simulink model "controlSystem"  (R2023a)
settings: Solver=FixedStepDiscrete  StartTime=0.0  StopTime=inf  FixedStep=T  RelTol=1e-3  EnableMultiTasking=on
PreLoadFcn:
  | T=0.01;
  | alpha=0.02;
undefined symbols (not defined in the file): DiscIntNeverNeededParam
libraries: arduinolib x2, slpidlib x2, spsFirstOrderFilterLib x1, simulink x1, arduinosensorlib x1, arduinowifilib x1
settings Model: ExtModeTrigDuration=2  Creator=michele  LastModifiedBy=root
settings SolverCC: AlgebraicLoopSolver=TrustRegion
settings OptimizationCC: EnhancedBackFolding=on  PassReuseOutputArgsAs=Individual arguments  ZeroExternalMemoryAtStartup=off  ZeroInternalMemoryAtStartup=off  MaxStackSize=64  OptimizeBlockOrder=speed  DifferentSizesBufferReuse=on  OptimizationCustomize=off  EfficientTunableParamExpr=on
settings DebuggingCC: ParameterTunabilityLossMsg=error
settings HardwareCC: ProdBitPerPointer=32  ProdBitPerSizeT=32  ProdBitPerPtrDiffT=32  ProdLargestAtomicInteger=Long  ProdLargestAtomicFloat=Double  ProdWordSize=32  ProdHWDeviceType=ARM Compatible->ARM Cortex  UseEmbeddedCoderFeatures=off  UseSimulinkCoderFeatures=off
settings SFSimCC: MATLABDynamicMemAlloc=off
settings RTWCC: Description=Embedded Coder  SystemTargetFile=ert.tlc  HardwareBoard=ESP32-WROOM(Arduino Compatible)  TLCOptions="-aInlineSetEventsForThisBaseRateFcn=TLC_FALSE -aSuppressMultiTaskScheduler=TLC_FALSE  -aRateBasedStepFcn=0"  TemplateMakefile=ert_default_tmf  Toolchain=ESP32  BuildConfiguration=Faster Runs  DLArmComputeVersion=19.05
settings CodeAppCC: ForceParamTrailComments=on  IgnoreCustomStorageClasses=off  OperatorAnnotations=on  SimulinkDataObjDesc=on  SFDataObjDesc=on  MangleLength=10  InsertBlockDesc=on
settings ERTTargetCC: SupportContinuousTime=on  SupportNonInlinedSFcns=on  SupportVariableSizeSignals=on  ExtModeTransport=3  ExtModeStaticAlloc=on  ExtModeAutomaticAllocSize=off  ExtModeStaticAllocSize=65536  ExtModeMexFile=ext_xcp  ExtModeIntrfLevel=Level2 - Open

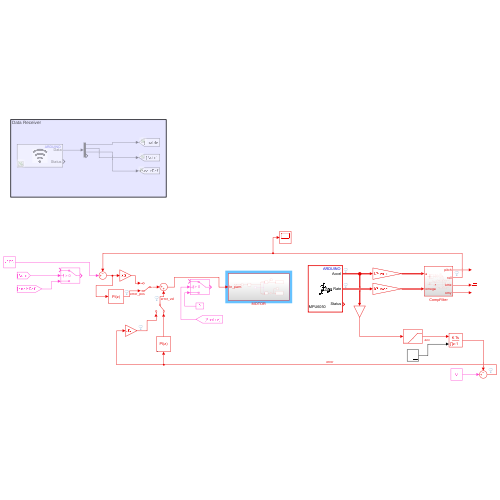
[thumbnail: Simulink's stored preview of the top-level diagram]
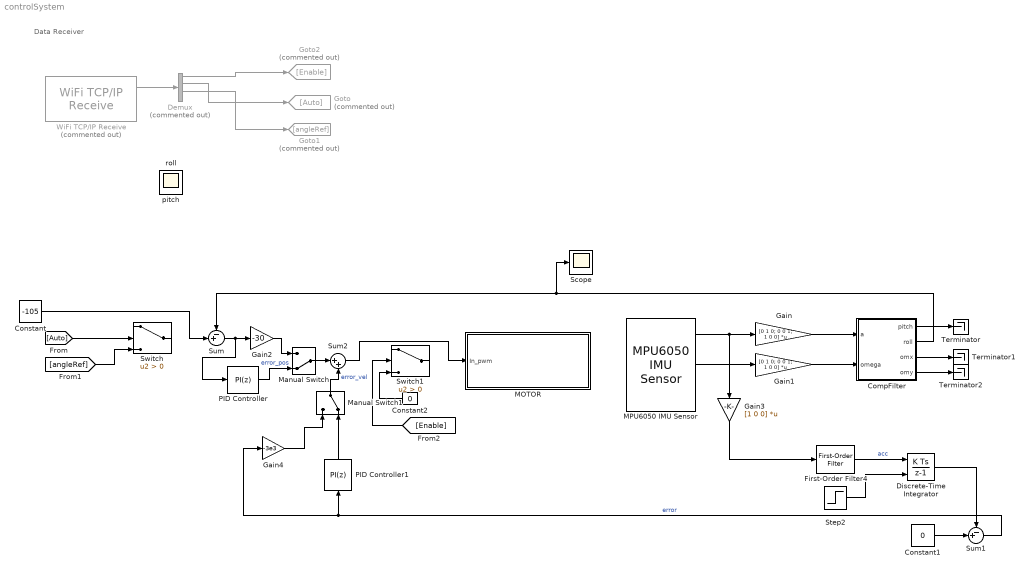
== system controlSystem ==
  note: Data Receiver
  CompFilter : Subsystem
  Constant : Constant  Value=-105
  Constant1 : Constant  Value=0
  Constant2 : Constant  Value=0
  Demux : Demux  Commented=on
  Discrete-Time Integrator : DiscreteIntegrator  ExternalReset=level  SampleTime=-1  ICPrevOutput=DiscIntNeverNeededParam  ICPrevScaledInput=DiscIntNeverNeededParam
  First-Order Filter4 : spsFirstOrderFilterLib/First-Order Filter  FilterType=Highpass  Tc=10e-3  Ts=0.01  Initialize=off  Vac_Init=[0, 0, 60]  Vdc_Init=0  PlotResponse=off  FreqRange="[0,  200,  1]"
  Gain : Gain  Gain=[0 1 0; 0 0 1; 1 0 0]  Multiplication=Matrix(K*u) (u vector)
  Gain1 : Gain  Gain=[0 1 0; 0 0 1; 1 0 0]  Multiplication=Matrix(K*u) (u vector)
  Gain2 : Gain  Gain=-30
  Gain3 : Gain  Gain=[1 0 0]  Multiplication=Matrix(K*u) (u vector)
  Gain4 : Gain  Gain=-3e3
  Goto : Goto  Commented=on  GotoTag=Auto
  Goto1 : Goto  Commented=on  GotoTag=angleRef
  Goto2 : Goto  Commented=on  GotoTag=Enable
  MOTOR : Subsystem
  MPU6050 IMU Sensor : arduinosensorlib/MPU6050 IMU Sensor  SlaveAddress=0x68  Accel=on  AngularRate=on  Temperature=off  Status=on  Timestamp=off  EulerAngles=off  Quat=off  AccelRange=2G  GyroRange=250 dps  DmpOdr=200 Hz  Dlpf=Accelerometer: 44Hz, Gyroscope: 42Hz  spf=1  SampleTime=-1  QueueSizeFactor=1
  Manual Switch : ManualSwitch  CurrentSetting=0
  Manual Switch1 : ManualSwitch  CurrentSetting=0
  PID Controller : slpidlib/PID Controller  Controller=PI  Form=Parallel  TimeDomain=Discrete-time  UseExternalTs=off  SampleTime=-1  IntegratorMethod=Forward Euler  FilterMethod=Forward Euler  ControllerParametersSource=internal  P=-4  I=-.3  UseKiTs=off  D=0  N=100  UseFilter=on  TunerSelectOption=Transfer Function Based (PID Tuner App)  InitialConditionSource=internal  InitialConditionForIntegrator=0  InitialConditionForFilter=0  DifferentiatorICPrevScaledInput=0  ExternalReset=none  TrackingMode=off  Kt=1  LimitOutput=off  SatLimitsSource=internal  UpperSaturationLimit=inf  LowerSaturationLimit=-inf  LinearizeAsGain=on  AntiWindupMode=none  Kb=1  LimitIntegrator=off  UpperIntegratorSaturationLimit=inf  LowerIntegratorSaturationLimit=-inf  POutMin=[]  POutMax=[]  IOutMin=[]  IOutMax=[]  DOutMin=[]  DOutMax=[]  NOutMin=[]  NOutMax=[]  SumOutMin=[]  SumOutMax=[]  SaturationOutMin=[]  SaturationOutMax=[]  PParamMin=[]  PParamMax=[]  IParamMin=[]  IParamMax=[]  DParamMin=[]  DParamMax=[]  NParamMin=[]  NParamMax=[]  KbParamMin=[]  KbParamMax=[]  KtParamMin=[]  KtParamMax=[]  KbOutMin=[]  KbOutMax=[]  KtOutMin=[]  KtOutMax=[]  IntegratorOutMin=[]  IntegratorOutMax=[]  FilterOutMin=[]  FilterOutMax=[]  SumI1OutMin=[]  SumI1OutMax=[]  SumI2OutMin=[]  SumI2OutMax=[]  SumI3OutMin=[]  SumI3OutMax=[]  SumI4OutMin=[]  SumI4OutMax=[]  SumDOutMin=[]  SumDOutMax=[]  DifferentiatorOutMin=[]  DifferentiatorOutMax=[]  FilterDiffOutCoefMin=[]  FilterDiffOutCoefMax=[]  ReciprocalOutMin=[]  ReciprocalOutMax=[]  SumDenOutMin=[]  SumDenOutMax=[]  SumNumOutMin=[]  SumNumOutMax=[]  DivideOutMin=[]  DivideOutMax=[]  UdiffTsProdOutMin=[]  UdiffTsProdOutMax=[]  NTsProdOutMin=[]  NTsProdOutMax=[]  UintegralTsProdOutMin=[]  UintegralTsProdOutMax=[]  UngainTsProdOutMin=[]  UngainTsProdOutMax=[]  ClampingZeroOutDataTypeStr=Inherit: Inherit via back propagation  ClampingZeroOutMin=[]  ClampingZeroOutMax=[]  FilterDenConstantOutDataTypeStr=Inherit: Inherit via back propagation  FilterDenConstantOutMin=[]  FilterDenConstantOutMax=[]  PCopyOutDataTypeStr=Inherit: Inherit via back propagation  PCopyOutMin=[]  PCopyOutMax=[]  NCopyOutDataTypeStr=Inherit: Inherit via back propagation  NCopyOutMin=[]  NCopyOutMax=[]  IntegratorContinuousStateAttributes=''  IntegratorStateMustResolveToSignalObject=off  IntegratorRTWStateStorageClass=Auto  FilterContinuousStateAttributes=''  FilterStateMustResolveToSignalObject=off  FilterRTWStateStorageClass=Auto  ParallelPVariant=InternalParameters  IdealPVariant=Disabled  IVariant=InternalParameters  DVariant=Disabled  IntegratorVariant=Discrete  SatVariant=Disabled  AWVariant=Passthrough  PCopyVariant=Disabled  TRVariant=Disabled  FdbkBlocksVariant=Forward  IdealPFdbkVariant=Disabled  SatFdbkVariant=Disabled  DerivativeFilterVariant=Disabled  NVariant=Disabled  NCopyVariant=Disabled_SignalSpec  FilterICVariant=Disabled  IntegratorICVariant=InternalICs  ExternalResetVariant=Disabled  TRSumVariant=Passthrough  SumFdbkVariant=Disabled  SumVariant=Sum_PI  TsampFilterVariant=InternalTs  TsampNgainVariant=Passthrough  TsampIntegralVariant=Disabled_SignalSpec  ExternalSaturationOutDataTypeStr=Inherit: Same as second input
  PID Controller1 : slpidlib/PID Controller  Controller=PI  Form=Parallel  TimeDomain=Discrete-time  UseExternalTs=off  SampleTime=-1  IntegratorMethod=Forward Euler  FilterMethod=Forward Euler  ControllerParametersSource=internal  P=-2e3  I=-3e2  UseKiTs=off  D=0  N=100  UseFilter=on  TunerSelectOption=Transfer Function Based (PID Tuner App)  InitialConditionSource=internal  InitialConditionForIntegrator=0  InitialConditionForFilter=0  DifferentiatorICPrevScaledInput=0  ExternalReset=none  TrackingMode=off  Kt=1  LimitOutput=off  SatLimitsSource=internal  UpperSaturationLimit=inf  LowerSaturationLimit=-inf  LinearizeAsGain=on  AntiWindupMode=none  Kb=1  LimitIntegrator=off  UpperIntegratorSaturationLimit=inf  LowerIntegratorSaturationLimit=-inf  POutMin=[]  POutMax=[]  IOutMin=[]  IOutMax=[]  DOutMin=[]  DOutMax=[]  NOutMin=[]  NOutMax=[]  SumOutMin=[]  SumOutMax=[]  SaturationOutMin=[]  SaturationOutMax=[]  PParamMin=[]  PParamMax=[]  IParamMin=[]  IParamMax=[]  DParamMin=[]  DParamMax=[]  NParamMin=[]  NParamMax=[]  KbParamMin=[]  KbParamMax=[]  KtParamMin=[]  KtParamMax=[]  KbOutMin=[]  KbOutMax=[]  KtOutMin=[]  KtOutMax=[]  IntegratorOutMin=[]  IntegratorOutMax=[]  FilterOutMin=[]  FilterOutMax=[]  SumI1OutMin=[]  SumI1OutMax=[]  SumI2OutMin=[]  SumI2OutMax=[]  SumI3OutMin=[]  SumI3OutMax=[]  SumI4OutMin=[]  SumI4OutMax=[]  SumDOutMin=[]  SumDOutMax=[]  DifferentiatorOutMin=[]  DifferentiatorOutMax=[]  FilterDiffOutCoefMin=[]  FilterDiffOutCoefMax=[]  ReciprocalOutMin=[]  ReciprocalOutMax=[]  SumDenOutMin=[]  SumDenOutMax=[]  SumNumOutMin=[]  SumNumOutMax=[]  DivideOutMin=[]  DivideOutMax=[]  UdiffTsProdOutMin=[]  UdiffTsProdOutMax=[]  NTsProdOutMin=[]  NTsProdOutMax=[]  UintegralTsProdOutMin=[]  UintegralTsProdOutMax=[]  UngainTsProdOutMin=[]  UngainTsProdOutMax=[]  ClampingZeroOutDataTypeStr=Inherit: Inherit via back propagation  ClampingZeroOutMin=[]  ClampingZeroOutMax=[]  FilterDenConstantOutDataTypeStr=Inherit: Inherit via back propagation  FilterDenConstantOutMin=[]  FilterDenConstantOutMax=[]  PCopyOutDataTypeStr=Inherit: Inherit via back propagation  PCopyOutMin=[]  PCopyOutMax=[]  NCopyOutDataTypeStr=Inherit: Inherit via back propagation  NCopyOutMin=[]  NCopyOutMax=[]  IntegratorContinuousStateAttributes=''  IntegratorStateMustResolveToSignalObject=off  IntegratorRTWStateStorageClass=Auto  FilterContinuousStateAttributes=''  FilterStateMustResolveToSignalObject=off  FilterRTWStateStorageClass=Auto  ParallelPVariant=InternalParameters  IdealPVariant=Disabled  IVariant=InternalParameters  DVariant=Disabled  IntegratorVariant=Discrete  SatVariant=Disabled  AWVariant=Passthrough  PCopyVariant=Disabled  TRVariant=Disabled  FdbkBlocksVariant=Forward  IdealPFdbkVariant=Disabled  SatFdbkVariant=Disabled  DerivativeFilterVariant=Disabled  NVariant=Disabled  NCopyVariant=Disabled_SignalSpec  FilterICVariant=Disabled  IntegratorICVariant=InternalICs  ExternalResetVariant=Disabled  TRSumVariant=Passthrough  SumFdbkVariant=Disabled  SumVariant=Sum_PI  TsampFilterVariant=InternalTs  TsampNgainVariant=Passthrough  TsampIntegralVariant=Disabled_SignalSpec  ExternalSaturationOutDataTypeStr=Inherit: Same as second input
  Scope : Scope
  Step2 : Step  Time=2  Before=1  After=0  SampleTime=0
  Sum : Sum  Inputs=-+|
  Sum1 : Sum  Inputs=-+|
  Sum2 : Sum  Inputs=|++
  Switch : Switch  Criteria=u2 > Threshold  SaturateOnIntegerOverflow=off  InputSameDT=off
  Switch1 : Switch  Criteria=u2 > Threshold  SaturateOnIntegerOverflow=off  InputSameDT=off
  Terminator : Terminator
  Terminator1 : Terminator
  Terminator2 : Terminator
  WiFi TCP/IP Receive : arduinowifilib/WiFi TCP//IP Receive  Commented=on  Mode_=Server  serverport=25000  RemoteAddr_=192.168.1.2  RemoteServerPort_=25000  DataType_=uint8  DataSize_=1  SampleTime_=0.1  remoteipoctet1=192  remoteipoctet2=168  remoteipoctet3=1  remoteipoctet4=2  wifiTCPServerIndex=0  wifiTCPClientIndex=0  blockPlatform=ARDUINO  isARMArch=false  SimulateUsing=Code generation  BlockingMode_=off  BlockTimeout_=0.1
  pitch : Scope
  roll : Scope
  wires:
  MPU6050 IMU Sensor/2 -> Gain1/1
  CompFilter/1(pitch) -> Terminator/1
  CompFilter/2(roll) -> Scope/1, Sum/1
  CompFilter/3(omx) -> Terminator1/1
  CompFilter/4(omy) -> Terminator2/1
  Gain/1 -> CompFilter/1(a)
  Gain1/1 -> CompFilter/2(omega)
  Gain2/1 -> Manual Switch/1
  Sum/1 -> PID Controller/1, Gain2/1
  PID Controller/1 -> Manual Switch/2  "error_pos"
  MPU6050 IMU Sensor/1 -> Gain/1, Gain3/1
  Discrete-Time Integrator/1 -> Sum1/1
  Step2/1 -> Discrete-Time Integrator/2
  First-Order Filter4/1 -> Discrete-Time Integrator/1  "acc"
  Gain3/1 -> First-Order Filter4/1
  Constant1/1 -> Sum1/2
  Sum1/1 -> Gain4/1, PID Controller1/1  "error"
  Manual Switch1/1 -> Sum2/2  "error_vel"
  Manual Switch/1 -> Sum2/1
  PID Controller1/1 -> Manual Switch1/2
  Gain4/1 -> Manual Switch1/1
  [Auto] -> Switch/2
  [angleRef] -> Switch/3
  Demux/3 -> Goto1/1
  WiFi TCP/IP Receive/1 -> Demux/1
  Demux/1 -> Goto2/1
  Demux/2 -> Goto/1
  Constant2/1 -> Switch1/3
  [Enable] -> Switch1/2
  Sum2/1 -> MOTOR/1(In_pwm)
  Constant/1 -> Sum/2

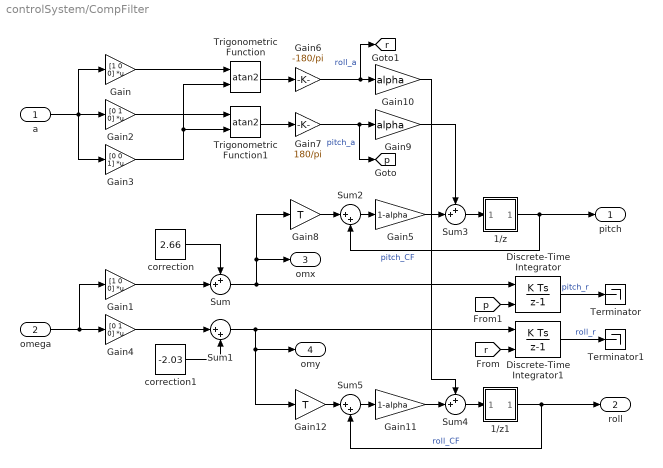
== system controlSystem/CompFilter ==
  a : Inport
  omega : Inport  Port=2
  1/z : Subsystem
  1/z1 : Subsystem
  Discrete-Time Integrator : DiscreteIntegrator  InitialConditionSource=external  SampleTime=-1  ICPrevOutput=DiscIntNeverNeededParam  ICPrevScaledInput=DiscIntNeverNeededParam
  Discrete-Time Integrator1 : DiscreteIntegrator  InitialConditionSource=external  SampleTime=-1  ICPrevOutput=DiscIntNeverNeededParam  ICPrevScaledInput=DiscIntNeverNeededParam
  Gain : Gain  Gain=[1 0 0]  Multiplication=Matrix(K*u)
  Gain1 : Gain  Gain=[1 0 0]  Multiplication=Matrix(K*u)
  Gain10 : Gain  Gain=alpha
  Gain11 : Gain  Gain=1-alpha
  Gain12 : Gain  Gain=T
  Gain2 : Gain  Gain=[0 1 0]  Multiplication=Matrix(K*u)
  Gain3 : Gain  Gain=[0 0 1]  Multiplication=Matrix(K*u)
  Gain4 : Gain  Gain=[0 1 0]  Multiplication=Matrix(K*u)
  Gain5 : Gain  Gain=1-alpha
  Gain6 : Gain  Gain=-180/pi
  Gain7 : Gain  Gain=180/pi
  Gain8 : Gain  Gain=T
  Gain9 : Gain  Gain=alpha
  Sum : Sum  Inputs=++|
  Sum1 : Sum  Inputs=|++
  Sum2 : Sum  Inputs=|++
  Sum3 : Sum  Inputs=++|
  Sum4 : Sum  Inputs=++|
  Sum5 : Sum  Inputs=|++
  Terminator : Terminator
  Terminator1 : Terminator
  Trigonometric Function : Trigonometry  Operator=atan2
  Trigonometric Function1 : Trigonometry  Operator=atan2
  correction : Constant  Value=2.66  SampleTime=T
  correction1 : Constant  Value=-2.03  SampleTime=T
  pitch : Outport
  roll : Outport  Port=2
  omx : Outport  Port=3
  omy : Outport  Port=4
  tag scope: p=global, r=global
  wires:
  a/1 -> Gain3/1, Gain2/1, Gain/1
  omega/1 -> Gain1/1, Gain4/1
  Trigonometric Function/1 -> Gain6/1
  Gain/1 -> Trigonometric Function/1
  Gain2/1 -> Trigonometric Function1/1
  Gain3/1 -> Trigonometric Function1/2, Trigonometric Function/2
  Trigonometric Function1/1 -> Gain7/1
  Discrete-Time Integrator1/1 -> Terminator1/1  "roll_r"
  Gain1/1 -> Sum/2
  Sum/1 -> Gain8/1, omx/1, Discrete-Time Integrator/1
  correction/1 -> Sum/1
  Gain4/1 -> Sum1/1
  correction1/1 -> Sum1/2
  Gain7/1 -> [p], Gain9/1  "pitch_a"
  Gain6/1 -> [r], Gain10/1  "roll_a"
  Sum2/1 -> Gain5/1
  Gain8/1 -> Sum2/1
  Gain9/1 -> Sum3/1
  1/z/1(out) -> pitch/1, Sum2/2  "pitch_CF"
  Gain5/1 -> Sum3/2
  Sum3/1 -> 1/z/1(in)
  Discrete-Time Integrator/1 -> Terminator/1  "pitch_r"
  1/z1/1(out) -> Sum5/2, roll/1  "roll_CF"
  Sum4/1 -> 1/z1/1(in)
  Gain11/1 -> Sum4/2
  Gain10/1 -> Sum4/1
  Sum1/1 -> omy/1, Gain12/1, Discrete-Time Integrator1/1
  Gain12/1 -> Sum5/1
  Sum5/1 -> Gain11/1
  [r] -> Discrete-Time Integrator1/2
  [p] -> Discrete-Time Integrator/2

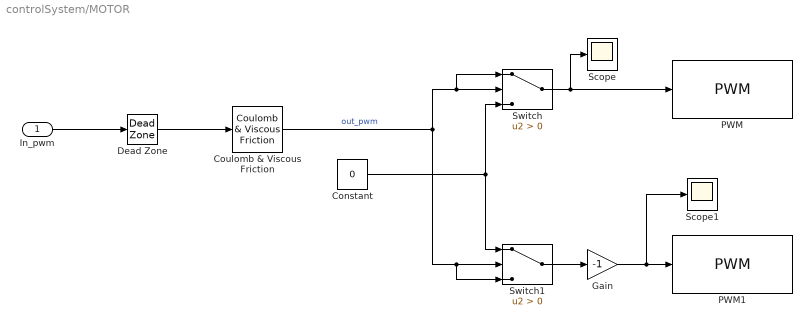
== system controlSystem/MOTOR ==
  In_pwm : Inport
  Constant : Constant  Value=0
  Coulomb & Viscous Friction : simulink/Discontinuities/Coulomb & Viscous Friction  offset=[180]  gain=1
  Dead Zone : DeadZone  LowerValue=-100  UpperValue=100
  Gain : Gain  Gain=-1
  PWM : arduinolib/PWM  pinNumber=32  frequencyType=Default  desiredFrequency=490.2  achievableFrequency=490.2
  PWM1 : arduinolib/PWM  pinNumber=33  frequencyType=Default  desiredFrequency=490.2  achievableFrequency=490.2
  Scope : Scope
  Scope1 : Scope
  Switch : Switch  Criteria=u2 > Threshold  SaturateOnIntegerOverflow=off  InputSameDT=off
  Switch1 : Switch  Criteria=u2 > Threshold  SaturateOnIntegerOverflow=off  InputSameDT=off
  wires:
  Switch1/1 -> Gain/1
  Gain/1 -> PWM1/1, Scope1/1
  Switch/1 -> Scope/1, PWM/1
  Constant/1 -> Switch1/1, Switch/3
  In_pwm/1 -> Dead Zone/1
  Coulomb & Viscous Friction/1 -> Switch1/2, Switch1/3, Switch/1, Switch/2  "out_pwm"
  Dead Zone/1 -> Coulomb & Viscous Friction/1

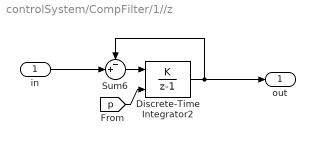
== system controlSystem/CompFilter/1//z ==
  in : Inport
  Discrete-Time Integrator2 : DiscreteIntegrator  IntegratorMethod=Accumulation: Forward Euler  InitialConditionSource=external  SampleTime=-1  ICPrevOutput=DiscIntNeverNeededParam  ICPrevScaledInput=DiscIntNeverNeededParam
  Sum6 : Sum  Inputs=-+|
  out : Outport
  wires:
  in/1 -> Sum6/2
  [p] -> Discrete-Time Integrator2/2
  Sum6/1 -> Discrete-Time Integrator2/1
  Discrete-Time Integrator2/1 -> out/1, Sum6/1

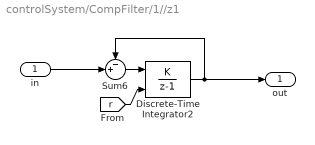
== system controlSystem/CompFilter/1//z1 ==
  in : Inport
  Discrete-Time Integrator2 : DiscreteIntegrator  IntegratorMethod=Accumulation: Forward Euler  InitialConditionSource=external  SampleTime=-1  ICPrevOutput=DiscIntNeverNeededParam  ICPrevScaledInput=DiscIntNeverNeededParam
  Sum6 : Sum  Inputs=-+|
  out : Outport
  wires:
  in/1 -> Sum6/2
  [r] -> Discrete-Time Integrator2/2
  Sum6/1 -> Discrete-Time Integrator2/1
  Discrete-Time Integrator2/1 -> out/1, Sum6/1
